simulink model "psb1phPWM"  (Simulink 6.0)
settings: Solver=VariableStepDiscrete  SolverMode=SingleTasking  StartTime=0.0  StopTime=0.1  MaxStep=Ts  RelTol=1e-3
PreLoadFcn:
  | assignin('base','Ts',[1/60/3240])
undefined symbols (not defined in the file or in its folder): Ts
libraries: powerlib2 x33, powerlib_extras x3
settings Model: Creator=patrice  LastModifiedBy=batserve  ExtModeTrigMode=oneshot  ExtModeArmWhenConnect=off  ExtModeAutoUpdateStatusClock=off
settings DataIOCC: LimitDataPoints=off  SignalLoggingName=sigsOut
settings OptimizationCC: BlockReduction=off  BooleanDataType=off
settings DebuggingCC: CheckExecutionContextPreStartOutputMsg=on  CheckExecutionContextRuntimeOutputMsg=on  SolverPrmCheckMsg=none
settings HardwareCC: TargetUnknown=on
settings RTWCC: TemplateMakefile=grt_unix.tmf

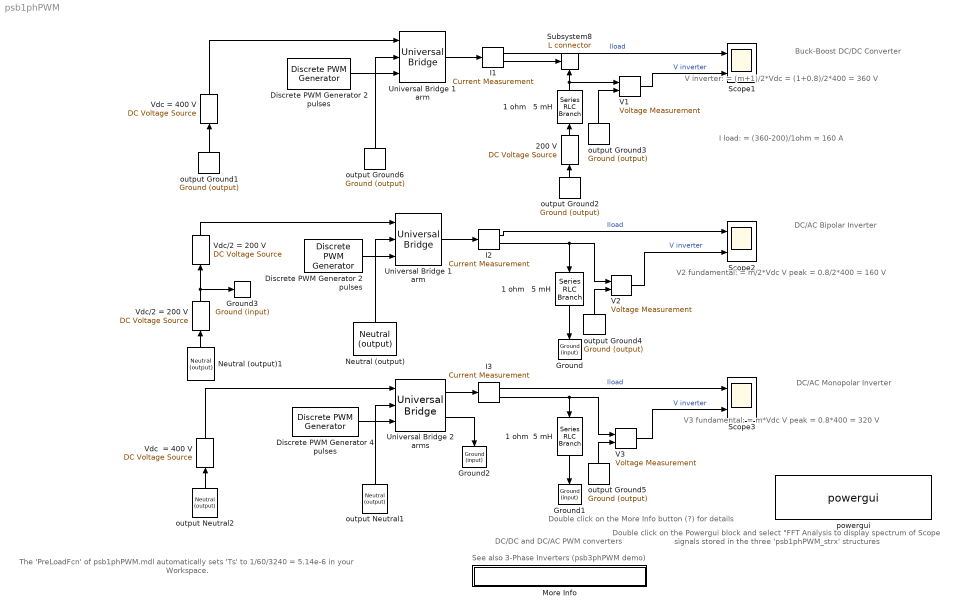
== system psb1phPWM ==
  note: V3 fundamental:
      | = m*Vdc V peak
      | = 0.8*400
      | = 320 V
  note: DC/DC and DC/AC PWM converters
  note: Double click on the More Info button (?) for details
  note: V2 fundamental:
      | = m/2*Vdc V peak
      | = 0.8/2*400
      | = 160 V
  note: V inverter:
      | = (m+1)/2*Vdc
      | = (1+0.8)/2*400
      | = 360 V
  note: See also 3-Phase Inverters (psb3phPWM demo)
  note: The 'PreLoadFcn' of psb1phPWM.mdl automatically
      | sets 'Ts' to 1/60/3240 = 5.14e-6 in your Workspace.
  note: Double click on the Powergui block and
      | select "FFT Analysis to display spectrum
      | of Scope  signals stored in the three
      | 'psb1phPWM_strx' structures
  note: Buck-Boost DC/DC Converter
  note: DC/AC Bipolar Inverter
  note: DC/AC Monopolar Inverter
  note: I load:
      | = (360-200)/1ohm
      | = 160 A
  1 ohm   5 mH : powerlib2/Elements/Series RLC Branch  Tag=PoWeRsYsTeMbLoCk  Orientation=down  a=1  b=5e-03  c=inf  mesure=None  PSBOutputType=1
  "1 ohm   5 mH  " : powerlib2/Elements/Series RLC Branch  Tag=PoWeRsYsTeMbLoCk  Orientation=up  a=1  b=5e-03  c=inf  mesure=None  PSBOutputType=1
  "1 ohm  5 mH " : powerlib2/Elements/Series RLC Branch  Tag=PoWeRsYsTeMbLoCk  Orientation=down  a=1  b=5e-03  c=inf  mesure=None  PSBOutputType=1
  200 V : powerlib2/Electrical Sources/DC Voltage Source  Tag=PoWeRsYsTeMbLoCk  Orientation=up  V=200  mesure=None  PSBOutputType=1
  Discrete PWM Generator 2 pulses : powerlib_extras/Discrete  Control Blocks/Discrete PWM Generator  GeneratorMode="1-arm  bridge (2 pulses)"  Fc=1080  Ts=Ts  Internal=on  mIndex=0.8  Freq=60  Phase=0
  "Discrete PWM Generator 2 pulses " : powerlib_extras/Discrete  Control Blocks/Discrete PWM Generator  GeneratorMode="1-arm  bridge (2 pulses)"  Fc=1080  Ts=Ts  Internal=on  mIndex=0.8  Freq=0  Phase=0
  Discrete PWM Generator 4 pulses : powerlib_extras/Discrete  Control Blocks/Discrete PWM Generator  GeneratorMode="2-arm  bridge (4 pulses)"  Fc=1080  Ts=Ts  Internal=on  mIndex=0.8  Freq=60  Phase=0
  Ground : powerlib2/Connectors/Ground (input)  Tag=PoWeRsYsTeMbLoCk  Orientation=down
  Ground1 : powerlib2/Connectors/Ground (input)  Tag=PoWeRsYsTeMbLoCk  Orientation=down
  Ground2 : powerlib2/Connectors/Ground (input)  Tag=PoWeRsYsTeMbLoCk  Orientation=down
  Ground3 : powerlib2/Connectors/Ground (input)  Tag=PoWeRsYsTeMbLoCk
  I1 : powerlib2/Measurements/Current Measurement  Tag=PoWeRsYsTeMmEaSuReMeNt  PhasorSimulation=off  OutputType=Magnitude  PSBOutputType=01  PSBequivalent=0
  I2 : powerlib2/Measurements/Current Measurement  Tag=PoWeRsYsTeMmEaSuReMeNt  PhasorSimulation=off  OutputType=Magnitude  PSBOutputType=01  PSBequivalent=0
  "I3 " : powerlib2/Measurements/Current Measurement  Tag=PoWeRsYsTeMmEaSuReMeNt  PhasorSimulation=off  OutputType=Magnitude  PSBOutputType=01  PSBequivalent=0
  More Info : Subsystem
      mask Display: disp('? : Double click here for more info')
  Neutral (output) : powerlib2/Connectors/Neutral (output)  Tag=PoWeRsYsTeMbLoCk  Orientation=up  no=2  PSBOutputType=1
  Neutral (output)1 : powerlib2/Connectors/Neutral (output)  Tag=PoWeRsYsTeMbLoCk  Orientation=up  no=2  PSBOutputType=1
  "Scope1 " : Scope  NumInputPorts=2
      settings: TimeRange=0.1  YMin=0~-50  YMax=175~400  SaveName=psb1phPWM1_str  MaxDataPoints=500000
  Scope2 : Scope  NumInputPorts=2
      settings: TimeRange=0.1  YMin=-100~-300  YMax=100~300  SaveName=psb1phPWM2_str  MaxDataPoints=500000
  Scope3 : Scope  NumInputPorts=2
      settings: TimeRange=0.1  YMin=-200~-500  YMax=200~500  SaveName=psb1phPWM3_str  MaxDataPoints=500000
  Subsystem8 : powerlib2/Connectors/L connector  Tag=PoWeRsYsTeMbLoCk  Orientation=up
  Universal Bridge 1 arm : powerlib2/Power Electronics/Universal Bridge  Tag=PoWeRsYsTeMbLoCk  arms=1  confi=ABC as output terminals  injcc=10000  cf=inf  device=IGBT / Diodes  Ron=1e-4  Lon=0  VFs="[  1  1  ]"  Vf=.8  gtoparameters=[ 10e-6 , 20e-6 ]  igbtparameters=[ 1e-6 , 2e-6 ]  mesure=None  PSBOutputType=111
  "Universal Bridge 1 arm " : powerlib2/Power Electronics/Universal Bridge  Tag=PoWeRsYsTeMbLoCk  arms=1  confi=ABC as output terminals  injcc=10000  cf=inf  device=IGBT / Diodes  Ron=1e-4  Lon=0  VFs="[  1  1  ]"  Vf=.8  gtoparameters=[ 10e-6 , 20e-6 ]  igbtparameters=[ 1e-6 , 2e-6 ]  mesure=None  PSBOutputType=111
  Universal Bridge 2 arms : powerlib2/Power Electronics/Universal Bridge  Tag=PoWeRsYsTeMbLoCk  arms=2  confi=ABC as output terminals  injcc=10000  cf=inf  device=IGBT / Diodes  Ron=1e-4  Lon=0  VFs="[  1  1  ]"  Vf=.8  gtoparameters=[ 10e-6 , 20e-6 ]  igbtparameters=[ 1e-6 , 2e-6 ]  mesure=None  PSBOutputType=111
  "V1 " : powerlib2/Measurements/Voltage Measurement  Tag=PoWeRsYsTeMmEaSuReMeNt  PhasorSimulation=off  OutputType=Magnitude  PSBOutputType=0  PSBequivalent=0
  V2 : powerlib2/Measurements/Voltage Measurement  Tag=PoWeRsYsTeMmEaSuReMeNt  PhasorSimulation=off  OutputType=Magnitude  PSBOutputType=0  PSBequivalent=0
  V3 : powerlib2/Measurements/Voltage Measurement  Tag=PoWeRsYsTeMmEaSuReMeNt  PhasorSimulation=off  OutputType=Magnitude  PSBOutputType=0  PSBequivalent=1
  "Vdc  = 400 V  " : powerlib2/Electrical Sources/DC Voltage Source  Tag=PoWeRsYsTeMbLoCk  Orientation=up  V=400  mesure=None  PSBOutputType=1
  Vdc = 400 V : powerlib2/Electrical Sources/DC Voltage Source  Tag=PoWeRsYsTeMbLoCk  Orientation=up  V=400  mesure=None  PSBOutputType=1
  Vdc/2 = 200 V : powerlib2/Electrical Sources/DC Voltage Source  Tag=PoWeRsYsTeMbLoCk  Orientation=up  V=200  mesure=None  PSBOutputType=1
  "Vdc/2 = 200 V " : powerlib2/Electrical Sources/DC Voltage Source  Tag=PoWeRsYsTeMbLoCk  Orientation=up  V=200  mesure=None  PSBOutputType=1
  output Ground{1..6} (6 alike) : powerlib2/Connectors/Ground (output)  Tag=PoWeRsYsTeMbLoCk  Orientation=up  PSBOutputType=1
  output Neutral1 : powerlib2/Connectors/Neutral (output)  Tag=PoWeRsYsTeMbLoCk  Orientation=up  no=3  PSBOutputType=1
  output Neutral2 : powerlib2/Connectors/Neutral (output)  Tag=PoWeRsYsTeMbLoCk  Orientation=up  no=3  PSBOutputType=1
  powergui : powerlib2/powergui  Frange=[0:2:500]  Ylog=off  Xlog=off  save=off  variable=ZData  structure=psb1phPWM1_str  ZoomFFT=on  StartTime=0.1-2/60  cycles=1  DisplayStyle=off  fundamental=60  FreqAxis=off  MaxFrequency=5000  frequencyindice=1  frequencyindicesteady=1  RmsSteady=1  display=off  Ts=Ts  methode=off  frequency=60  echomessages=off
  wires:
  I1/1 -> "Scope1 "/1  "Iload"
  Universal Bridge 1 arm/1 -> I1/1
  "Discrete PWM Generator 2 pulses "/1 -> Universal Bridge 1 arm/3
  Vdc = 400 V/1 -> Universal Bridge 1 arm/1
  I2/1 -> Scope2/1  "Iload"
  "Universal Bridge 1 arm "/1 -> I2/1
  Discrete PWM Generator 2 pulses/1 -> "Universal Bridge 1 arm "/3
  V2/1 -> Scope2/2  "V inverter"
  Vdc/2 = 200 V/1 -> "Universal Bridge 1 arm "/1
  I2/2 -> 1 ohm   5 mH/1, V2/1
  "Vdc/2 = 200 V "/1 -> Vdc/2 = 200 V/1, Ground3/1
  Neutral (output)1/1 -> "Vdc/2 = 200 V "/1
  Discrete PWM Generator 4 pulses/1 -> Universal Bridge 2 arms/3
  Universal Bridge 2 arms/1 -> "I3 "/1
  "I3 "/1 -> Scope3/1  "Iload"
  "I3 "/2 -> "1 ohm  5 mH "/1, V3/1
  V3/1 -> Scope3/2  "V inverter"
  Universal Bridge 2 arms/2 -> Ground2/1
  "Vdc  = 400 V  "/1 -> Universal Bridge 2 arms/1
  output Neutral2/1 -> "Vdc  = 400 V  "/1
  "V1 "/1 -> "Scope1 "/2  "V inverter"
  output Ground1/1 -> Vdc = 400 V/1
  I1/2 -> Subsystem8/Enable
  200 V/1 -> "1 ohm   5 mH  "/1
  output Ground2/1 -> 200 V/1
  "1 ohm   5 mH  "/1 -> Subsystem8/1, "V1 "/1
  output Ground3/1 -> "V1 "/2
  1 ohm   5 mH/1 -> Ground/1
  output Ground4/1 -> V2/2
  "1 ohm  5 mH "/1 -> Ground1/1
  output Ground5/1 -> V3/2
  output Ground6/1 -> Universal Bridge 1 arm/2
  Neutral (output)/1 -> "Universal Bridge 1 arm "/2
  output Neutral1/1 -> Universal Bridge 2 arms/2

== system psb1phPWM/More Info ==
  note: G. Sybille and P. Giroux (Hydro-Quebec)
  note: Demonstration
  note: Circuit Description
  note: This demonstration illustrates use of the Universal Bridge and
      | Discrete PWM Pulse Generator blocks. It also demonstrates
      | harmonic analysis of PWM waveforms using the Powergui/FFT tool.
  note: The system consists of three independant circuits illustrating various PWM DC/DC and DC/AC inverters.
      | All converters are controlled in open loop with the Discrete PWM Generator block available in the Extras/Discrete Control Blocks library.
      | The three circuits use the same DC voltage (Vdc = 400V), carrier frequency (1080 Hz) and modulation index (m = 0.8) .
      | From top to bottom, the three circuits are:
      |
      | 1. DC/DC, two-quadrant converter (one-arm; two-switches)
      | 2. DC/AC,  bipolar converter  (one-arm; two-switches)
      | 3. DC/AC, monopolar  converter (two-arms; four-switches)
      |
      | In order to allow further signal processing, signals displayed on the three Scope blocks  (sampled at simulation sampling rate of 3240 samples/cycle)
      | are stored in three  variables named 'psb1phPWM1_str' , 'psb1phPWM2_str'  and  'psb1phPWM3_str'  (structures with time).
  note: Run the simulation and observe the following two waveforms on the Scope blocks:
      | current into the load (trace 1), voltage generated by the PWM inverter (trace 2).
      |
      | Once the  simulation is completed, open the Powergui and select 'FFT Analysis' to display the 0 - 5000 Hz frequency spectrum of signals saved
      | in the three 'psb1phPWMx_str' structures. The FFT will be performed on  a 2-cycle window starting at t = 0.1 - 2/60 (last 2 cycles of recording).
      | For each circuit selelect Input labeled 'V inverter' . Click on Display and observe the frequency spectrum of last 2 cycles.
      |
      | The fundamental component of  V inverter (DC component in case of circuit 1) is displayed above the spectrum window.
      | Compare the magnitude of the fundamental or DC component of the inverter voltage with the theoretical values given in the  circuit.
      | Compare also the harmonic contents in the inverter voltage for the two-switch and four-switch DC/AC inverters.
      |
      | For the two-switch inverter,  the first harmonics  occur around the carrier frequency (1080 Hz +- k*60 Hz, with a maximum of 103% at 1080 Hz ),
      | whereas for the four-switch inverter harmonics are lower and appear at double of carrier frequency (maximum of 40% at 2*1080+-60 Hz)
      | As a result, the current is "cleaner" for the four-switch inverter.
      | If you now perform a FFT on the signal Iload you will notice that the THD of load current is 7.3% for the two-switch inverter as compared to
      | only  2% for the four-switch inverter.
